simulink model "Fourier_Series_Sim"  (R2018b)
settings: Solver=FixedStepAuto  StartTime=0.0  StopTime=3*T  FixedStep=0.01  RelTol=1e-3  EnableMultiTasking=on
values from neighbouring files (symbols this model uses):
  amp = 5    [Fourier_Series_Mat.m]    (also in bode_test_001.mat; bode_test_002.mat; bode_test_003.mat; bode_test_004.mat)
  T = ps(k)    [Fourier_Series_Mat.m]    (also in bode_test_001.mat = 1; bode_test_002.mat = 1; bode_test_003.mat = 0.1; bode_test_004.mat = 0.1)
libraries: arduinolib x2
settings Model: ExtModeTrigDuration=2  Creator=FV  LastModifiedBy=alessandrosebastianelli
settings OptimizationCC: EnhancedBackFolding=on  PassReuseOutputArgsAs=Individual arguments  MaxStackSize=64  OptimizeBlockOrder=speed  DifferentSizesBufferReuse=on  OptimizationCustomize=off
settings DebuggingCC: ParameterTunabilityLossMsg=error
settings HardwareCC: ProdBitPerInt=16  ProdBitPerPointer=16  ProdBitPerSizeT=16  ProdBitPerPtrDiffT=16  ProdLargestAtomicFloat=None  ProdWordSize=8  ProdHWDeviceType=Atmel->AVR  UseEmbeddedCoderFeatures=off  UseSimulinkCoderFeatures=off
settings SFSimCC: SimUseLocalCustomCode=off  MATLABDynamicMemAlloc=off
settings RTWCC: SystemTargetFile=ert.tlc  HardwareBoard=Arduino Mega 2560  TemplateMakefile=ert_default_tmf  GenerateReport=on  RTWUseLocalCustomCode=off  Toolchain=Arduino AVR  BuildConfiguration=Faster Runs  IncludeHyperlinkInReport=on  LaunchReport=on  GenerateTraceInfo=on  GenerateTraceReport=on  GenerateTraceReportSl=on  GenerateTraceReportSf=on  GenerateTraceReportEml=on
settings CodeAppCC: ForceParamTrailComments=on  IgnoreCustomStorageClasses=off  OperatorAnnotations=on  SimulinkDataObjDesc=on  SFDataObjDesc=on  InsertBlockDesc=on
settings ERTTargetCC: SupportContinuousTime=on  SupportNonInlinedSFcns=on  SupportVariableSizeSignals=on

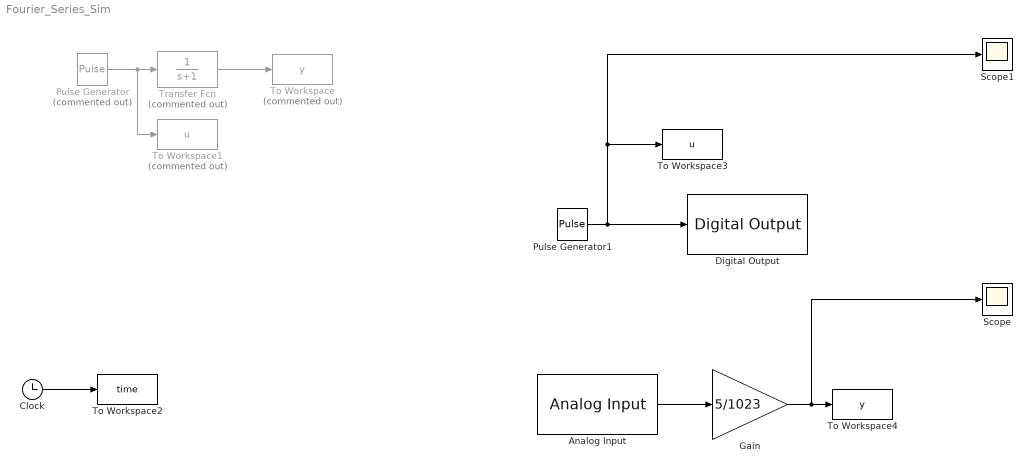
== system Fourier_Series_Sim ==
  Analog Input : arduinolib/Analog Input  pinNumber=0  ReadResultsOnly=off  ConversionTriggerSource=Software  ExternalTriggerType=uint32(0)  OutputDataType=uint16  EnableConversionCompleteNotify=off  EnableOuputStatus=off  SampleTime=-1  blockPlatform=arduino
  Clock : Clock
  Digital Output : arduinolib/Digital Output  pinNumber=7  blockPlatform=arduino
  Gain : Gain  Gain=5/1023  OutDataTypeStr=double
  Pulse Generator : DiscretePulseGenerator  Commented=on  PulseType=Time based  Amplitude=amp  Period=T  PulseWidth=50
  Pulse Generator1 : DiscretePulseGenerator  PulseType=Time based  Amplitude=amp  Period=T  PulseWidth=50
  Scope : Scope
  Scope1 : Scope
  To Workspace : ToWorkspace  Commented=on  VariableName=y  SampleTime=-1
      settings: Save2DSignal=2-D array (concatenate along first dimension)
  To Workspace1 : ToWorkspace  Commented=on  VariableName=u  SampleTime=-1
      settings: Save2DSignal=2-D array (concatenate along first dimension)
  To Workspace2 : ToWorkspace  VariableName=time  SampleTime=-1
      settings: Save2DSignal=2-D array (concatenate along first dimension)
  To Workspace3 : ToWorkspace  VariableName=u  SampleTime=-1
      settings: Save2DSignal=2-D array (concatenate along first dimension)
  To Workspace4 : ToWorkspace  VariableName=y  SampleTime=-1
      settings: Save2DSignal=2-D array (concatenate along first dimension)
  Transfer Fcn : TransferFcn  Commented=on  Denominator=[1 1]
  wires:
  Transfer Fcn/1 -> To Workspace/1
  Pulse Generator/1 -> To Workspace1/1, Transfer Fcn/1
  Clock/1 -> To Workspace2/1
  Pulse Generator1/1 -> Scope1/1, To Workspace3/1, Digital Output/1
  Analog Input/1 -> Gain/1
  Gain/1 -> Scope/1, To Workspace4/1
